simulink model "saveFLC"  (R2019a)
settings: Solver=VariableStepAuto  StartTime=0.0  StopTime=10.0  RelTol=1e-3
values from neighbouring files (symbols this model uses):
  Bm = 0.0022    [State_of_Art.m]    (also in results_plotter_one_run20.m)
  Jm = 0.0004    [State_of_Art.m]    (also in results_plotter_one_run20.m)
  Kb = 0.05    [State_of_Art.m]    (also in results_plotter_one_run20.m)
  Kt = 0.015    [State_of_Art.m]    (also in results_plotter_one_run20.m)
  La = 2.7    [State_of_Art.m]    (also in results_plotter_one_run20.m)
  Ra = 0.4    [State_of_Art.m]    (also in results_plotter_one_run20.m)
libraries: fuzblock x1
settings Model: Creator=Nelson Manuel  LastModifiedBy=Nelson Manuel

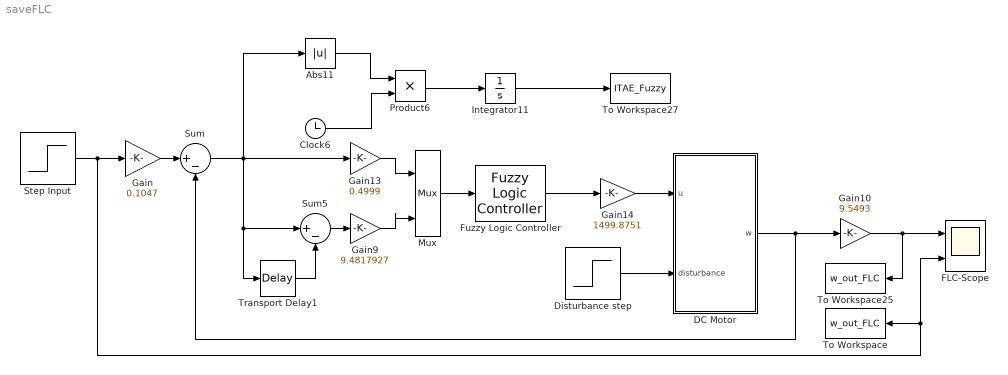
== system saveFLC ==
  Abs11 : Abs
  Clock6 : Clock
  DC Motor : Subsystem
  Disturbance step : Step  Time=0  After=0.01  SampleTime=0
  FLC-Scope : Scope  NumInputPorts=2
  Fuzzy Logic Controller : fuzblock/Fuzzy Logic  Controller  FIS=FLC_Controller_updated  OutputSampleNumber=101  DataType=double  FuzzifiedInputs=off  RuleFiringStrengths=off  RuleOutputs=off  AggregatedOutputs=off  SimulateUsing=Interpreted execution  OutOfRangeInputValueMessage=none  NoRuleFiredMessage=none  EmptyOutputFuzzySetMessage=none
  Gain : Gain  Gain=0.1047
  Gain10 : Gain  Gain=9.5493
  Gain13 : Gain  Gain=0.4999
  Gain14 : Gain  Gain=1499.8751
  Gain9 : Gain  Gain=9.4817927
  Integrator11 : Integrator
  Mux : Mux  Inputs=2
  Product6 : Product
  Step Input : Step  Time=0  SampleTime=0
  Sum : Sum  Inputs=|+-
  Sum5 : Sum  Inputs=|+-
  To Workspace : ToWorkspace  VariableName=w_out_FLC  SaveFormat=Timeseries  SampleTime=-1
  To Workspace25 : ToWorkspace  VariableName=w_out_FLC  SaveFormat=Timeseries  SampleTime=-1
  To Workspace27 : ToWorkspace  VariableName=ITAE_Fuzzy  SaveFormat=Timeseries  SampleTime=-1
  Transport Delay1 : TransportDelay  DelayTime=0.00056797432  BufferSize=2048
  wires:
  Sum/1 -> Transport Delay1/1, Sum5/1, Gain13/1, Abs11/1
  DC Motor/1(w) -> Gain10/1, Sum/2
  Sum5/1 -> Gain9/1
  Product6/1 -> Integrator11/1
  Gain13/1 -> Mux/1
  Gain9/1 -> Mux/2
  Clock6/1 -> Product6/2
  Abs11/1 -> Product6/1
  Step Input/1 -> To Workspace/1, FLC-Scope/2, Gain/1
  Disturbance step/1 -> DC Motor/2(disturbance)
  Integrator11/1 -> To Workspace27/1
  Gain/1 -> Sum/1
  Transport Delay1/1 -> Sum5/2
  Mux/1 -> Fuzzy Logic Controller/1
  Gain10/1 -> FLC-Scope/1, To Workspace25/1
  Fuzzy Logic Controller/1 -> Gain14/1
  Gain14/1 -> DC Motor/1(u)

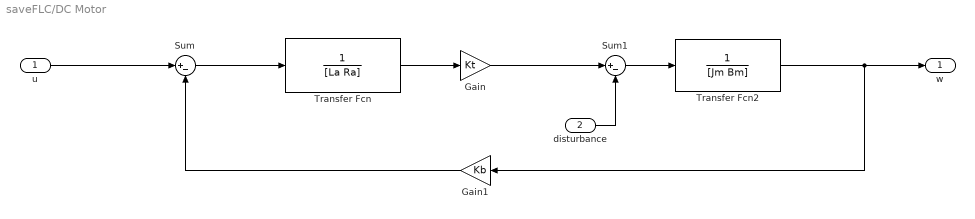
== system saveFLC/DC Motor ==
  u : Inport
  disturbance : Inport  Port=2
  Gain : Gain  Gain=Kt
  Gain1 : Gain  Gain=Kb
  Sum : Sum  Inputs=|+-
  Sum1 : Sum  Inputs=|+-
  Transfer Fcn : TransferFcn  Denominator=[La Ra]
  Transfer Fcn2 : TransferFcn  Denominator=[Jm Bm]
  w : Outport
  wires:
  Sum/1 -> Transfer Fcn/1
  Transfer Fcn2/1 -> w/1, Gain1/1
  disturbance/1 -> Sum1/2
  Gain/1 -> Sum1/1
  Gain1/1 -> Sum/2
  u/1 -> Sum/1
  Transfer Fcn/1 -> Gain/1
  Sum1/1 -> Transfer Fcn2/1
